simulink model "exercise_3c"  (R2018a)
settings: Solver=VariableStepAuto  StartTime=0.0  StopTime=10.0  RelTol=1e-3
undefined symbols (not defined in the file or in its folder): p
settings Model: Creator=mz-171742  LastModifiedBy=mz-171742

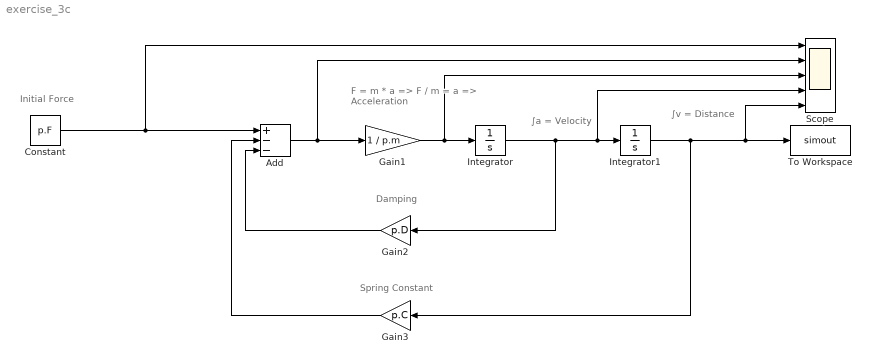
== system exercise_3c ==
  note: Initial Force
  note: Spring Constant
  note: Damping
  note: ∫v = Distance
  note: F = m * a
      | => F / m = a
      | => Acceleration
  note: ∫a = Velocity
  Add : Sum  Inputs=+--
  Constant : Constant  Value=p.F
  Gain1 : Gain  Gain=1 / p.m
  Gain2 : Gain  Gain=p.D
  Gain3 : Gain  Gain=p.C
  Integrator : Integrator
  Integrator1 : Integrator
  Scope : Scope  NumInputPorts=5
  To Workspace : ToWorkspace  VariableName=simout  SaveFormat=Structure With Time  SampleTime=-1
  wires:
  Constant/1 -> Scope/1, Add/1
  Add/1 -> Scope/2, Gain1/1
  Gain1/1 -> Scope/3, Integrator/1
  Integrator/1 -> Gain2/1, Scope/4, Integrator1/1
  Gain2/1 -> Add/3
  Integrator1/1 -> Gain3/1, Scope/5, To Workspace/1
  Gain3/1 -> Add/2
